simulink model "untitled"  (R2020a)
settings: Solver=VariableStepAuto  StartTime=0.0  StopTime=20  RelTol=1e-6
undefined symbols (not defined in the file or in its folder): B, f, K, M
settings Model: PacingRate=0.001000  Creator=faith  LastModifiedBy=faith

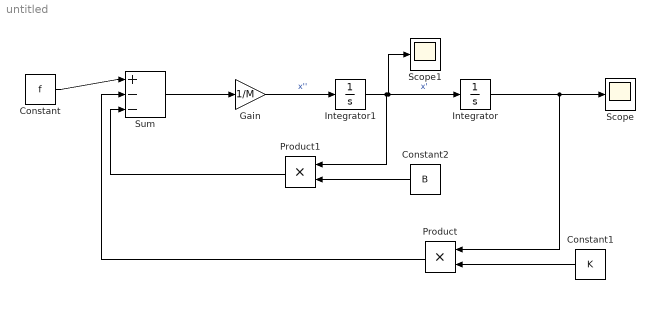
== system untitled ==
  Constant : Constant  Value=f
  Constant1 : Constant  Value=K
  Constant2 : Constant  Value=B
  Gain : Gain  Gain=1/M
  Integrator : Integrator
  Integrator1 : Integrator
  Product : Product
  Product1 : Product
  Scope : Scope
  Scope1 : Scope
  Sum : Sum  Inputs=|+--
  wires:
  Integrator/1 -> Scope/1, Product/1
  Integrator1/1 -> Product1/1, Integrator/1, Scope1/1  "x'"
  Gain/1 -> Integrator1/1  "x''"
  Constant/1 -> Sum/1
  Constant1/1 -> Product/2
  Product/1 -> Sum/2
  Constant2/1 -> Product1/2
  Product1/1 -> Sum/3
  Sum/1 -> Gain/1
